simulink model "MotorModelo6v"  (R2021a)
settings: Solver=VariableStepAuto  StartTime=0.0  StopTime=9  RelTol=1e-3
values from neighbouring files (symbols this model uses):
  B = p0(2)    [DC_Motor.m]    (also in Parametros_Motor.m = 0.002235795)
  J = p0(1)    [DC_Motor.m]    (also in Parametros_Motor.m = 0.000400955)
  Ka = p0(3)    [DC_Motor.m]    (also in Parametros_Motor.m = 0.23351629)
  Km = p0(4)    [DC_Motor.m]    (also in Parametros_Motor.m = 0.23351629)
  L = p0(6)    [DC_Motor.m]    (also in Parametros_Motor.m = 0.0015)
  R = p0(5)    [DC_Motor.m]    (also in Parametros_Motor.m = 3.4)
  Vm = 3.57    [Parametros_Motor.m]    (also in Regresion_Modelo.m)
undefined symbols (not defined in the file or in its folder): LF
libraries: instrumentseriallib x3, cstblocks x1
settings Model: Creator=Sergio  LastModifiedBy=Sergio
settings SolverCC: AlgebraicLoopSolver=TrustRegion
settings DataIOCC: ReturnWorkspaceOutputs=off
settings DebuggingCC: SFMachineParentedDataDiag=warning  ArithmeticOperatorsInVariantConditions=warning
settings SFSimCC: SimUseLocalCustomCode=off  CustomCodeUndefinedFunction=UseInterfaceOnly
settings RTWCC: RTWUseLocalCustomCode=off

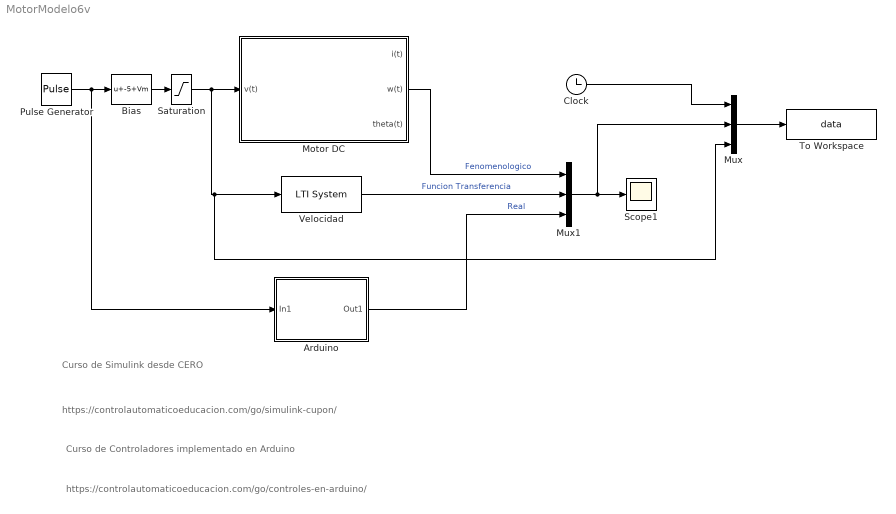
== system MotorModelo6v ==
  note: https://controlautomaticoeducacion.com/go/controles-en-arduino/
  note: Curso de Simulink desde CERO
  note: Curso de Controladores implementado en Arduino
  note: https://controlautomaticoeducacion.com/go/simulink-cupon/
  Arduino : Subsystem
  Bias : Bias  Bias=-5+Vm
  Clock : Clock
  Motor DC : Subsystem
  Mux : Mux  Inputs=3
  Mux1 : Mux  Inputs=3
  Pulse Generator : DiscretePulseGenerator  PulseType=Time based  Amplitude=5  Period=4  PulseWidth=50  PhaseDelay=2
  Saturation : Saturate  UpperLimit=5  LowerLimit=0
  Scope1 : Scope
  To Workspace : ToWorkspace  VariableName=data  SampleTime=0.05
  Velocidad : cstblocks/LTI System  sys=Gwv  IC=[]
  wires:
  Arduino/1(Out1) -> Mux1/3  "Real"
  Motor DC/2(w(t)) -> Mux1/1  "Fenomenologico"
  Velocidad/1 -> Mux1/2  "Funcion Transferencia"
  Bias/1 -> Saturation/1
  Saturation/1 -> Mux/3, Velocidad/1, Motor DC/1(v(t))
  Mux/1 -> To Workspace/1
  Clock/1 -> Mux/1
  Mux1/1 -> Mux/2, Scope1/1
  Pulse Generator/1 -> Bias/1, Arduino/1(In1)

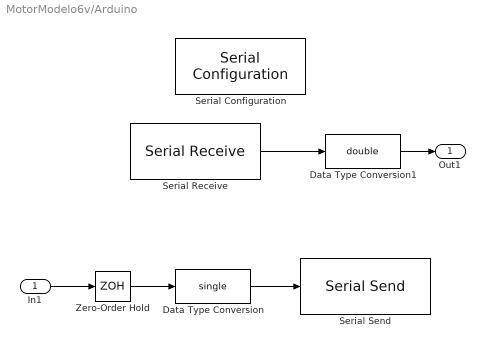
== system MotorModelo6v/Arduino ==
  In1 : Inport
  Data Type Conversion : DataTypeConversion  OutDataTypeStr=single
  Data Type Conversion1 : DataTypeConversion  OutDataTypeStr=double
  Serial Configuration : instrumentseriallib/Serial Configuration  Priority=-200000  Port=COM1  ComPort=COM1  BaudRate=9600  DataBits=8  Parity=none  StopBits=1  ByteOrder=little-endian  FlowControl=none  Timeout=10  SimulateUsing=Interpreted execution  BlockInModel=on
  Serial Receive : instrumentseriallib/Serial Receive  Priority=1  Port=COM1  ComPort=COM1  DataType=single  SaveDataType=uint8  ToggleHeader=on  Header='V'  ToggleTerminator=on  Terminator=LF ('\n')  CustomTerminator=[]  ToggleDataSize=on  DataSize=[1 1]  EnableBlockingMode=on  ActionDataUnavailable=Output last received value  ActionWhenDataUnavailable=Output last received value  CustomValue=0  SampleTime=0.05  SimulateUsing=Interpreted execution  BlockInModel=on
  Serial Send : instrumentseriallib/Serial Send  Priority=1  Port=COM1  ComPort=COM1  Header=[]  Terminator=<none>  CustomTerminator=[]  EnableBlockingMode=on  SimulateUsing=Interpreted execution  BlockInModel=on
  Zero-Order Hold : ZeroOrderHold  SampleTime=0.05
  Out1 : Outport
  wires:
  Serial Receive/1 -> Data Type Conversion1/1
  Data Type Conversion/1 -> Serial Send/1
  Zero-Order Hold/1 -> Data Type Conversion/1
  In1/1 -> Zero-Order Hold/1
  Data Type Conversion1/1 -> Out1/1

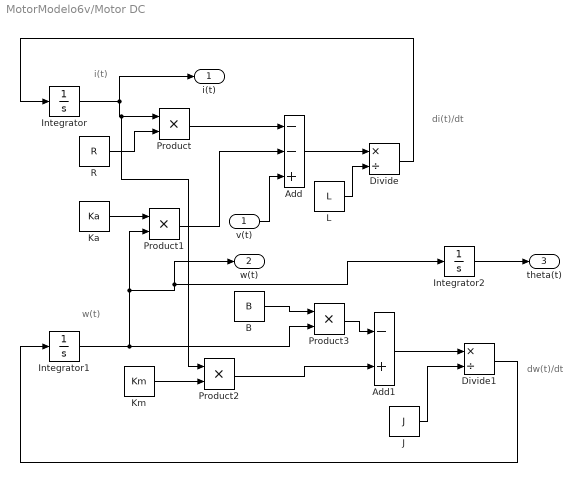
== system MotorModelo6v/Motor DC ==
  note: i(t)
  note: w(t)
  note: di(t)/dt
  note: dw(t)/dt
  v(t) : Inport
  Add : Sum  Inputs=--+
  Add1 : Sum  Inputs=-+
  B : Constant  Value=B
  Divide : Product  Inputs=*/
  Divide1 : Product  Inputs=*/
  Integrator : Integrator
  Integrator1 : Integrator
  Integrator2 : Integrator
  J : Constant  Value=J
  Ka : Constant  Value=Ka
  Km : Constant  Value=Km
  L : Constant  Value=L
  Product{,1..3} (4 alike) : Product
  R : Constant  Value=R
  i(t) : Outport  VectorParamsAs1DForOutWhenUnconnected=off
  w(t) : Outport  Port=2  VectorParamsAs1DForOutWhenUnconnected=off
  theta(t) : Outport  Port=3  VectorParamsAs1DForOutWhenUnconnected=off
  wires:
  Divide/1 -> Integrator/1
  Integrator/1 -> i(t)/1, Product2/1, Product/1
  Integrator1/1 -> Product3/2, w(t)/1, Integrator2/1, Product1/2
  R/1 -> Product/2
  Add1/1 -> Divide1/1
  v(t)/1 -> Add/3
  Ka/1 -> Product1/1
  J/1 -> Divide1/2
  Product3/1 -> Add1/1
  Product1/1 -> Add/2
  Add/1 -> Divide/1
  Product/1 -> Add/1
  L/1 -> Divide/2
  Divide1/1 -> Integrator1/1
  Integrator2/1 -> theta(t)/1
  B/1 -> Product3/1
  Km/1 -> Product2/2
  Product2/1 -> Add1/2
